simulink model "Filter100Tap"  (R2023a)
settings: Solver=VariableStepAuto  StartTime=0.0  StopTime=10.0  RelTol=1e-3
settings Model: Creator=nievep  LastModifiedBy=nievep

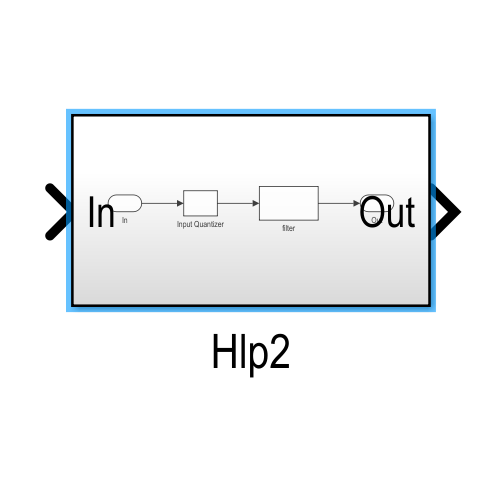
[thumbnail: Simulink's stored preview of the top-level diagram]
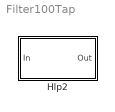
== system Filter100Tap ==
  Hlp2 : Subsystem  Tag=BlockMethodSubSystem

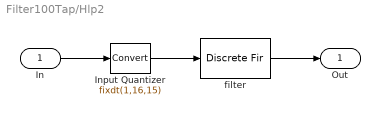
== system Filter100Tap/Hlp2 ==
  In : Inport
  Input Quantizer : DataTypeConversion  OutDataTypeStr=fixdt(1,16,15)  RndMeth=Round
  filter : DiscreteFir  Coefficients=[-0.000170997522781424883 -0.000882452135913848359 -0.00239994656804773301 -0.00531058374007885824 -0.00995485747537816143 -0.0165070159197606356 -0.024647142325532112 -0.0335047585109664453 -0.0416449438245579187 -0.0472913317629712962 -0.0487074067896422561 -0.0446961234849298991 -0.0350666289248854554 -0.0209146508663910179 -0.00457794152247266006 0.0107877765088917228 0.0219514990406600718 0.0264879945633294325 0.0235383321609250913 0.0141902242143751196 0.00130552827934083348 -0.0112153906365519921 -0.0195557884247666118 -0.02116380087169328 -0.015608259514624731 -0.00479703576565462808 0.00756719870514859731 0.0171680933770829991 0.0205350908725058928 0.0162965260444333515 0.00577221011630036154 -0.00735147480692063988 -0.018218060975501521 -0.0225065764821523774 -0.0180750057223073475 -0.0059417007351911565 0.00980706128525421841 0.0232477159072457668 0.0286521658483380841 0.0226735418481430161 0.00592513860107248252 -0.016660401777194165 -0.0369328615335007479 -0.0458492692814336938 -0.0363496092295966453 -0.00588050206011811374 0.042280514213420807 0.0994049437036765293 0.153379551385673357 0.191900023398869662 0.205857861146160809 0.191900023398869662 0.153379551385673357 0.0994049437036765293 0.042280514213420807 -0.00588050206011811374 -0.0363496092295966453 -0.0458492692814336938 -0.0369328615335007479 -0.016660401777194165 0.00592513860107248252 0.0226735418481430161 0.0286521658483380841 0.0232477159072457668 0.00980706128525421841 -0.0059417007351911565 -0.0180750057223073475 -0.0225065764821523774 -0.018218060975501521 -0.00735147480692063988 0.00577221011630036154 0.0162965260444333515 0.0205350908725058928 0.0171680933770829991 0.00756719870514859731 -0.00479703576565462808 -0.015608259514624731 -0.02116380087169328 -0.0195557884247666118 -0.0112153906365519921 0.00130552827934083348 0.0141902242143751196 0.0235383321609250913 0.0264879945633294325 0.0219514990406600718 0.0107877765088917228 -0.00457794152247266006 -0.0209146508663910179 -0.0350666289248854554 -0.0446961234849298991 -0.0487074067896422561 -0.0472913317629712962 -0.0416449438245579187 -0.0335047585109664453 -0.024647142325532112 -0.0165070159197606356 -0.00995485747537816143 -0.00531058374007885824 -0.00239994656804773301 -0.000882452135913848359 -0.000170997522781424883]  InputProcessing=Columns as channels (frame based)  CoefDataTypeStr=fixdt(true,16,17)  ProductDataTypeStr=fixdt(true,31,32)  AccumDataTypeStr=fixdt(true,35,32)  OutDataTypeStr=fixdt(true,35,32)  RndMeth=Convergent
  Out : Outport
  wires:
  In/1 -> Input Quantizer/1
  Input Quantizer/1 -> filter/1
  filter/1 -> Out/1
